simulink model "Q6_c_joint_space_solution"  (R2017a)
settings: Solver=FixedStepAuto  StartTime=0.0  StopTime=10.0  FixedStep=0.01  RelTol=0.00001
model workspace (MAT data in the model file):
  Kp_1 = 10000
  Kp_2 = 10000
  Kv_1 = 200
  Kv_2 = 200
  a_1 = 1
  a_2 = 1
  g = 9.8
  m_1 = 1
  m_2 = 1
  theta_d_dot = 1
  theta_d_double_dot = 1
libraries: simulink x3
settings Model: Creator=Omer  LastModifiedBy=Omer
settings ModelReferenceCC: ModelReferenceMinAlgLoopOccurrences=on

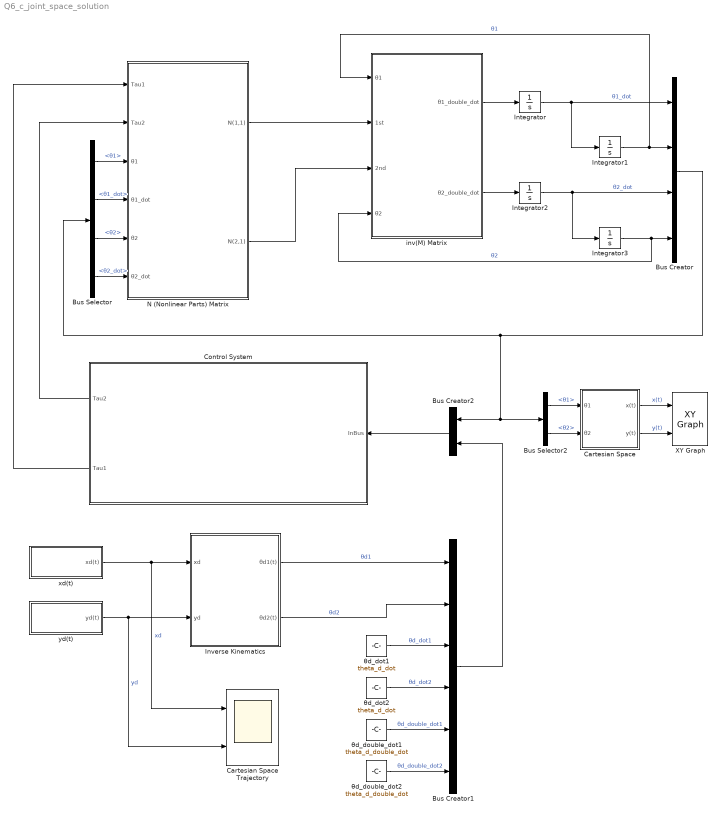
== system Q6_c_joint_space_solution ==
  Bus Creator : BusCreator  Inputs=4
  Bus Creator1 : BusCreator  Inputs=6
  Bus Creator2 : BusCreator  Inputs=2
  Bus Selector : BusSelector  OutputSignals=θ1,θ1_dot,θ2,θ2_dot
  Bus Selector2 : BusSelector  OutputSignals=θ1,θ2
  "Cartesian Space " : Subsystem  TreatAsAtomicUnit=on
  Cartesian Space Trajectory : Scope  NumInputPorts=2
  Control System : Subsystem  TreatAsAtomicUnit=on
  Integrator{,1..3} (4 alike) : Integrator
  Inverse Kinematics : Subsystem  TreatAsAtomicUnit=on
  N (Nonlinear Parts) Matrix : Subsystem  TreatAsAtomicUnit=on
  XY Graph : simulink/Sinks/XY Graph  xmin=-1  xmax=3  ymin=-1  ymax=2  st=-1
  inv(M) Matrix : Subsystem  TreatAsAtomicUnit=on
  xd(t) : Subsystem  TreatAsAtomicUnit=on
  yd(t) : Subsystem  TreatAsAtomicUnit=on
  θd_dot1 : Constant  Value=theta_d_dot
  θd_dot2 : Constant  Value=theta_d_dot
  θd_double_dot1 : Constant  Value=theta_d_double_dot
  θd_double_dot2 : Constant  Value=theta_d_double_dot
  wires:
  N (Nonlinear Parts) Matrix/2(N(2,1)) -> inv(M) Matrix/3(2nd)
  N (Nonlinear Parts) Matrix/1(N(1,1)) -> inv(M) Matrix/2(1st)
  Bus Creator/1 -> Bus Selector2/1, Bus Creator2/1, Bus Selector/1
  inv(M) Matrix/2(θ2_double_dot) -> Integrator2/1
  Bus Selector/1 -> N (Nonlinear Parts) Matrix/3("θ1 ")  "<θ1>"
  Integrator2/1 -> Integrator3/1, Bus Creator/3  "θ2_dot"
  Integrator3/1 -> inv(M) Matrix/4(θ2), Bus Creator/4  "θ2"
  Integrator1/1 -> inv(M) Matrix/1(θ1), Bus Creator/2  "θ1"
  Bus Selector/3 -> N (Nonlinear Parts) Matrix/5(θ2)  "<θ2>"
  Bus Selector/2 -> N (Nonlinear Parts) Matrix/4(θ1_dot)  "<θ1_dot>"
  Integrator/1 -> Bus Creator/1, Integrator1/1  "θ1_dot"
  Bus Selector/4 -> N (Nonlinear Parts) Matrix/6(θ2_dot)  "<θ2_dot>"
  inv(M) Matrix/1(θ1_double_dot) -> Integrator/1
  Bus Selector2/1 -> "Cartesian Space "/1(θ1)  "<θ1>"
  Bus Selector2/2 -> "Cartesian Space "/2(θ2)  "<θ2>"
  "Cartesian Space "/1(x(t)) -> XY Graph/1  "x(t)"
  "Cartesian Space "/2(y(t)) -> XY Graph/2  "y(t)"
  Bus Creator2/1 -> Control System/1(InBus)
  Bus Creator1/1 -> Bus Creator2/2
  θd_dot1/1 -> Bus Creator1/3  "θd_dot1"
  θd_dot2/1 -> Bus Creator1/4  "θd_dot2"
  θd_double_dot1/1 -> Bus Creator1/5  "θd_double_dot1"
  θd_double_dot2/1 -> Bus Creator1/6  "θd_double_dot2"
  xd(t)/1(xd(t)) -> Inverse Kinematics/1(xd), Cartesian Space Trajectory/1  "xd"
  yd(t)/1(yd(t)) -> Inverse Kinematics/2(yd), Cartesian Space Trajectory/2  "yd"
  Control System/1(Tau2) -> N (Nonlinear Parts) Matrix/2(Tau2)
  Control System/2(Tau1) -> N (Nonlinear Parts) Matrix/1(Tau1)
  Inverse Kinematics/1(θd1(t)) -> Bus Creator1/1  "θd1"
  Inverse Kinematics/2(θd2(t)) -> Bus Creator1/2  "θd2"

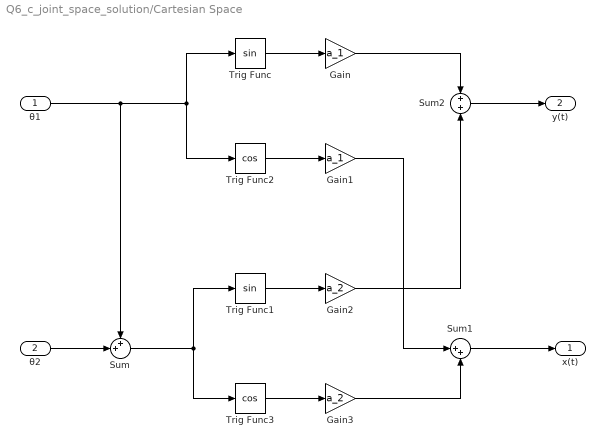
== system Q6_c_joint_space_solution/Cartesian Space  ==
  θ1 : Inport
  θ2 : Inport  Port=2
  Gain : Gain  Gain=a_1
  Gain1 : Gain  Gain=a_1
  Gain2 : Gain  Gain=a_2
  Gain3 : Gain  Gain=a_2
  Sum : Sum  Inputs=++|
  Sum1 : Sum  Inputs=|++
  Sum2 : Sum  Inputs=+|+
  Trig Func : Trigonometry
  Trig Func1 : Trigonometry
  Trig Func2 : Trigonometry  Operator=cos
  Trig Func3 : Trigonometry  Operator=cos
  x(t) : Outport
  y(t) : Outport  Port=2
  wires:
  θ1/1 -> Trig Func2/1, Trig Func/1, Sum/1
  θ2/1 -> Sum/2
  Sum/1 -> Trig Func3/1, Trig Func1/1
  Sum2/1 -> y(t)/1
  Sum1/1 -> x(t)/1
  Trig Func/1 -> Gain/1
  Gain/1 -> Sum2/1
  Trig Func2/1 -> Gain1/1
  Gain1/1 -> Sum1/1
  Trig Func1/1 -> Gain2/1
  Gain2/1 -> Sum2/2
  Trig Func3/1 -> Gain3/1
  Gain3/1 -> Sum1/2

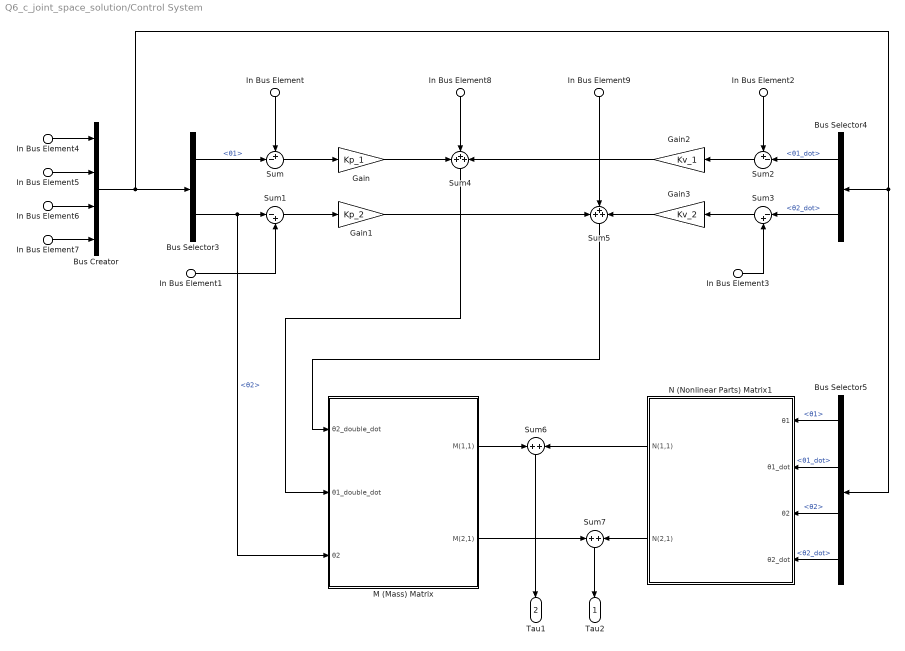
== system Q6_c_joint_space_solution/Control System ==
  In Bus Element : Inport  PortName=InBus  Element=signal2.θd1
  In Bus Element1 : Inport  PortName=InBus  Element=signal2.θd2
  In Bus Element2 : Inport  PortName=InBus  Element=signal2.θd_dot1
  In Bus Element3 : Inport  PortName=InBus  Element=signal2.θd_dot2
  In Bus Element8 : Inport  PortName=InBus  Element=signal2.θd_double_dot1
  In Bus Element9 : Inport  PortName=InBus  Element=signal2.θd_double_dot2
  In Bus Element4 : Inport  PortName=InBus  Element=signal1.θ1_dot
  In Bus Element5 : Inport  PortName=InBus  Element=signal1.θ1
  In Bus Element6 : Inport  PortName=InBus  Element=signal1.θ2_dot
  In Bus Element7 : Inport  PortName=InBus  Element=signal1.θ2
  Bus Creator : BusCreator  Inputs=4
  Bus Selector3 : BusSelector  OutputSignals=θ1,θ2
  Bus Selector4 : BusSelector  OutputSignals=θ1_dot,θ2_dot
  Bus Selector5 : BusSelector  OutputSignals=θ1,θ1_dot,θ2,θ2_dot
  Gain : Gain  Gain=Kp_1
  Gain1 : Gain  Gain=Kp_2
  Gain2 : Gain  Gain=Kv_1
  Gain3 : Gain  Gain=Kv_2
  M (Mass) Matrix : Subsystem  TreatAsAtomicUnit=on
  N (Nonlinear Parts) Matrix1 : Subsystem  TreatAsAtomicUnit=on
  Sum : Sum  Inputs=+-|
  Sum1 : Sum  Inputs=|-+
  Sum2 : Sum  Inputs=+-|
  Sum3 : Sum  Inputs=|-+
  Sum4 : Sum  Inputs=+++
  Sum5 : Sum  Inputs=+++
  Sum6 : Sum  Inputs=+|+
  Sum7 : Sum  Inputs=+|+
  Tau2 : Outport
  Tau1 : Outport  Port=2
  wires:
  Sum4/1 -> M (Mass) Matrix/2(θ1_double_dot)
  M (Mass) Matrix/1(M(1,1)) -> Sum6/1
  In Bus Element1/1 -> Sum1/2
  Sum7/1 -> Tau2/1
  In Bus Element7/1 -> Bus Creator/4
  In Bus Element3/1 -> Sum3/2
  N (Nonlinear Parts) Matrix1/1(N(1,1)) -> Sum6/2
  In Bus Element5/1 -> Bus Creator/2
  Gain1/1 -> Sum5/1
  In Bus Element4/1 -> Bus Creator/1
  Sum3/1 -> Gain3/1
  Sum2/1 -> Gain2/1
  In Bus Element2/1 -> Sum2/1
  Bus Selector5/2 -> N (Nonlinear Parts) Matrix1/2(θ1_dot)  "<θ1_dot>"
  Sum/1 -> Gain/1
  Bus Selector5/3 -> N (Nonlinear Parts) Matrix1/3(θ2)  "<θ2>"
  Sum5/1 -> M (Mass) Matrix/1(θ2_double_dot)
  M (Mass) Matrix/2(M(2,1)) -> Sum7/1
  Bus Selector5/4 -> N (Nonlinear Parts) Matrix1/4(θ2_dot)  "<θ2_dot>"
  Bus Selector4/1 -> Sum2/2  "<θ1_dot>"
  Sum6/1 -> Tau1/1
  Gain/1 -> Sum4/1
  In Bus Element8/1 -> Sum4/2
  In Bus Element9/1 -> Sum5/2
  Bus Selector5/1 -> N (Nonlinear Parts) Matrix1/1("θ1 ")  "<θ1>"
  Gain2/1 -> Sum4/3
  In Bus Element6/1 -> Bus Creator/3
  In Bus Element/1 -> Sum/1
  Gain3/1 -> Sum5/3
  Bus Selector3/2 -> M (Mass) Matrix/3(θ2), Sum1/1  "<θ2>"
  Bus Selector3/1 -> Sum/2  "<θ1>"
  N (Nonlinear Parts) Matrix1/2(N(2,1)) -> Sum7/2
  Bus Selector4/2 -> Sum3/1  "<θ2_dot>"
  Sum1/1 -> Gain1/1
  Bus Creator/1 -> Bus Selector3/1, Bus Selector4/1, Bus Selector5/1

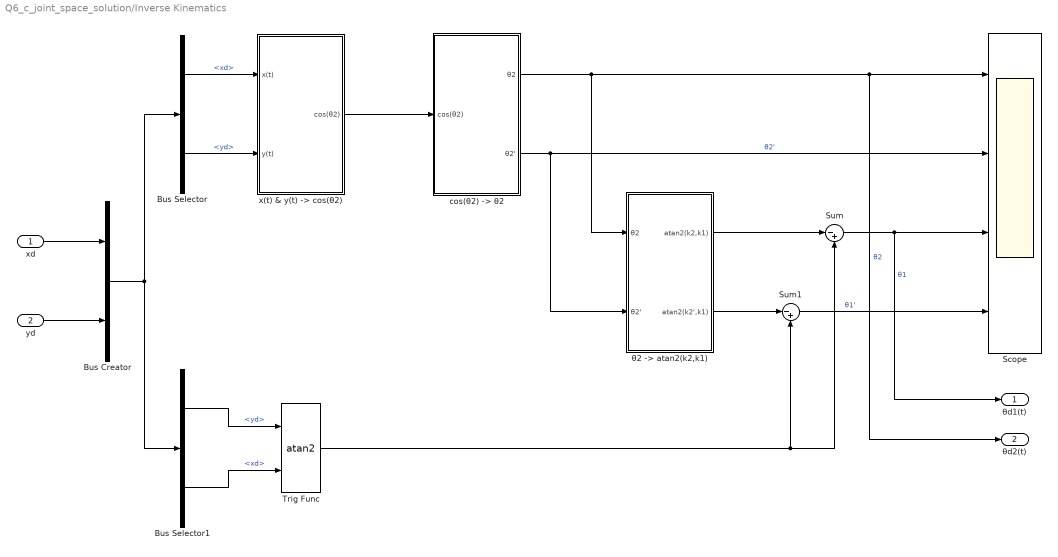
== system Q6_c_joint_space_solution/Inverse Kinematics ==
  xd : Inport
  yd : Inport  Port=2
  Bus Creator : BusCreator  Inputs=2
  Bus Selector : BusSelector  OutputSignals=xd,yd
  Bus Selector1 : BusSelector  OutputSignals=yd,xd
  Scope : Scope  NumInputPorts=4
  Sum : Sum  Inputs=|-+
  Sum1 : Sum  Inputs=|-+
  Trig Func : Trigonometry  Operator=atan2
  "cos(θ2) -> θ2" : Subsystem  TreatAsAtomicUnit=on
  "x(t) & y(t) -> cos(θ2)" : Subsystem  TreatAsAtomicUnit=on
  "θ2 -> atan2(k2,k1) " : Subsystem  TreatAsAtomicUnit=on
  θd1(t) : Outport
  θd2(t) : Outport  Port=2
  wires:
  Sum/1 -> θd1(t)/1, Scope/3  "θ1"
  Bus Selector/1 -> "x(t) & y(t) -> cos(θ2)"/1(x(t))  "<xd>"
  Bus Selector1/1 -> Trig Func/1  "<yd>"
  Sum1/1 -> Scope/4  "θ1'"
  "θ2 -> atan2(k2,k1) "/1(atan2(k2,k1)) -> Sum/1
  "θ2 -> atan2(k2,k1) "/2(atan2(k2',k1)) -> Sum1/1
  "x(t) & y(t) -> cos(θ2)"/1(cos(θ2)) -> "cos(θ2) -> θ2"/1(cos(θ2))
  Bus Selector1/2 -> Trig Func/2  "<xd>"
  Bus Creator/1 -> Bus Selector1/1, Bus Selector/1
  "cos(θ2) -> θ2"/1(θ2) -> "θ2 -> atan2(k2,k1) "/1(θ2), θd2(t)/1, Scope/1  "θ2"
  Bus Selector/2 -> "x(t) & y(t) -> cos(θ2)"/2(y(t))  "<yd>"
  Trig Func/1 -> Sum/2, Sum1/2
  "cos(θ2) -> θ2"/2(θ2') -> "θ2 -> atan2(k2,k1) "/2(θ2'), Scope/2  "θ2'"
  xd/1 -> Bus Creator/1
  yd/1 -> Bus Creator/2

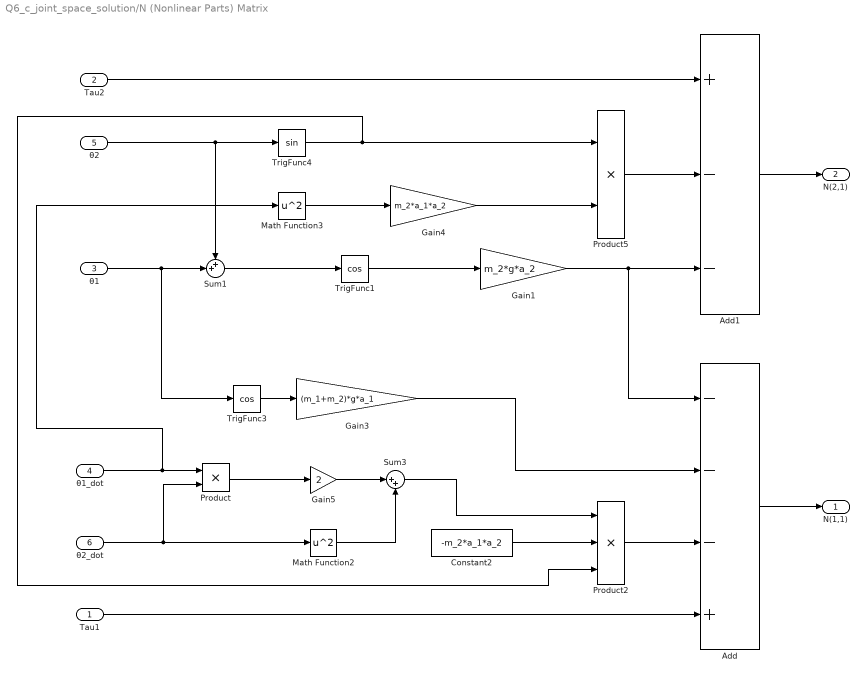
== system Q6_c_joint_space_solution/N (Nonlinear Parts) Matrix ==
  Tau1 : Inport
  Tau2 : Inport  Port=2
  "θ1 " : Inport  Port=3
  θ1_dot : Inport  Port=4
  θ2 : Inport  Port=5
  θ2_dot : Inport  Port=6
  Add : Sum  Inputs=---+
  Add1 : Sum  Inputs=+--
  Constant2 : Constant  Value=-m_2*a_1*a_2
  Gain1 : Gain  Gain=m_2*g*a_2
  Gain3 : Gain  Gain=(m_1+m_2)*g*a_1
  Gain4 : Gain  Gain=m_2*a_1*a_2
  Gain5 : Gain  Gain=2
  Math Function2 : Math  Operator=square  SaturateOnIntegerOverflow=on
  Math Function3 : Math  Operator=square  SaturateOnIntegerOverflow=on
  Product : Product
  Product2 : Product  Inputs=3
  Product5 : Product
  Sum1 : Sum  Inputs=++|
  Sum3 : Sum  Inputs=|++
  TrigFunc1 : Trigonometry  Operator=cos
  TrigFunc3 : Trigonometry  Operator=cos
  TrigFunc4 : Trigonometry
  N(1,1) : Outport
  N(2,1) : Outport  Port=2
  wires:
  Product2/1 -> Add/3
  Gain3/1 -> Add/2
  θ2/1 -> TrigFunc4/1, Sum1/1
  TrigFunc4/1 -> Product2/3, Product5/1
  Add1/1 -> N(2,1)/1
  Math Function3/1 -> Gain4/1
  θ1_dot/1 -> Product/1, Math Function3/1
  θ2_dot/1 -> Product/2, Math Function2/1
  Sum1/1 -> TrigFunc1/1
  Add/1 -> N(1,1)/1
  Sum3/1 -> Product2/1
  Math Function2/1 -> Sum3/2
  Tau2/1 -> Add1/1
  Constant2/1 -> Product2/2
  TrigFunc3/1 -> Gain3/1
  TrigFunc1/1 -> Gain1/1
  "θ1 "/1 -> TrigFunc3/1, Sum1/2
  Product5/1 -> Add1/2
  Tau1/1 -> Add/4
  Gain4/1 -> Product5/2
  Gain1/1 -> Add1/3, Add/1
  Product/1 -> Gain5/1
  Gain5/1 -> Sum3/1

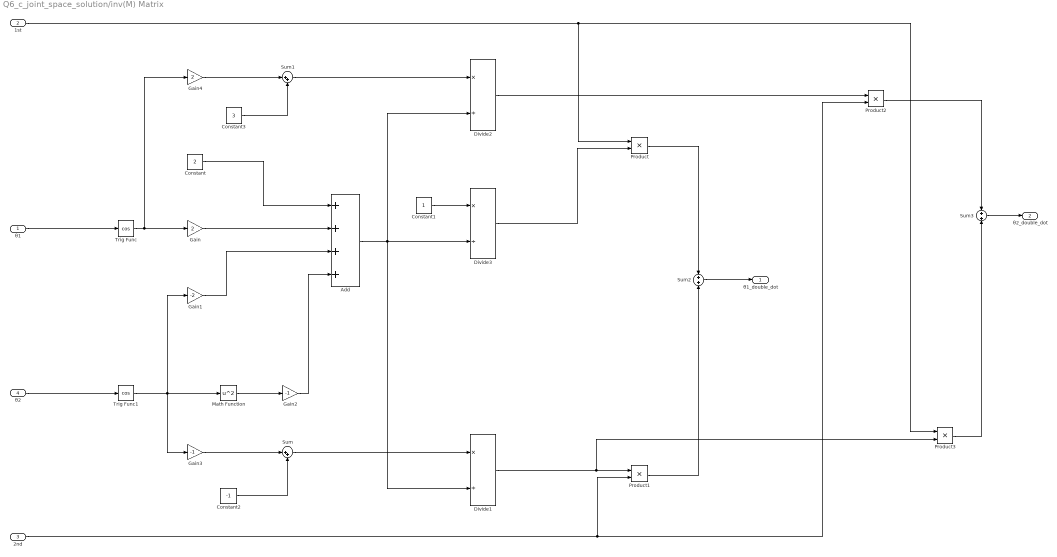
== system Q6_c_joint_space_solution/inv(M) Matrix ==
  θ1 : Inport
  1st : Inport  Port=2
  2nd : Inport  Port=3
  θ2 : Inport  Port=4
  Add : Sum  Inputs=4
  Constant : Constant  Value=2
  Constant1 : Constant
  Constant2 : Constant  Value=-1
  Constant3 : Constant  Value=3
  Divide1 : Product  Inputs=*/
  Divide2 : Product  Inputs=*/
  Divide3 : Product  Inputs=*/
  Gain : Gain  Gain=2
  Gain1 : Gain  Gain=-2
  Gain2 : Gain  Gain=-1
  Gain3 : Gain  Gain=-1
  Gain4 : Gain  Gain=2
  Math Function : Math  Operator=square  SaturateOnIntegerOverflow=on
  Product{,1..3} (4 alike) : Product
  Sum : Sum  Inputs=|++
  Sum1 : Sum  Inputs=|++
  Sum2 : Sum  Inputs=+|+
  Sum3 : Sum  Inputs=+|+
  Trig Func : Trigonometry  Operator=cos
  Trig Func1 : Trigonometry  Operator=cos
  θ1_double_dot : Outport
  θ2_double_dot : Outport  Port=2
  wires:
  Add/1 -> Divide2/2, Divide3/2, Divide1/2
  θ1/1 -> Trig Func/1
  θ2/1 -> Trig Func1/1
  Trig Func1/1 -> Gain3/1, Gain1/1, Math Function/1
  Trig Func/1 -> Gain4/1, Gain/1
  Constant/1 -> Add/1
  Gain/1 -> Add/2
  Gain1/1 -> Add/3
  Constant1/1 -> Divide3/1
  Math Function/1 -> Gain2/1
  Gain2/1 -> Add/4
  Gain3/1 -> Sum/1
  Constant2/1 -> Sum/2
  Sum/1 -> Divide1/1
  Constant3/1 -> Sum1/2
  Gain4/1 -> Sum1/1
  1st/1 -> Product/1, Product3/1
  Divide3/1 -> Product/2
  Divide1/1 -> Product3/2, Product1/1
  2nd/1 -> Product2/2, Product1/2
  Product/1 -> Sum2/1
  Product1/1 -> Sum2/2
  Sum2/1 -> θ1_double_dot/1
  Sum1/1 -> Divide2/1
  Divide2/1 -> Product2/1
  Product2/1 -> Sum3/1
  Sum3/1 -> θ2_double_dot/1
  Product3/1 -> Sum3/2

== system Q6_c_joint_space_solution/xd(t) ==
  Constant : Constant  Value=2
  Product : Product  Inputs=3
  Ramp : simulink/Sources/Ramp  slope=1  start=0  X0=0
  Step : Step  Time=0  SampleTime=0
  Step1 : Step  Time=2  Before=1  After=0  SampleTime=0
  Sum : Sum  Inputs=+-|
  xd(t) : Outport
  wires:
  Product/1 -> xd(t)/1
  Step/1 -> Product/2
  Step1/1 -> Product/3
  Constant/1 -> Sum/1
  Ramp/1 -> Sum/2
  Sum/1 -> Product/1

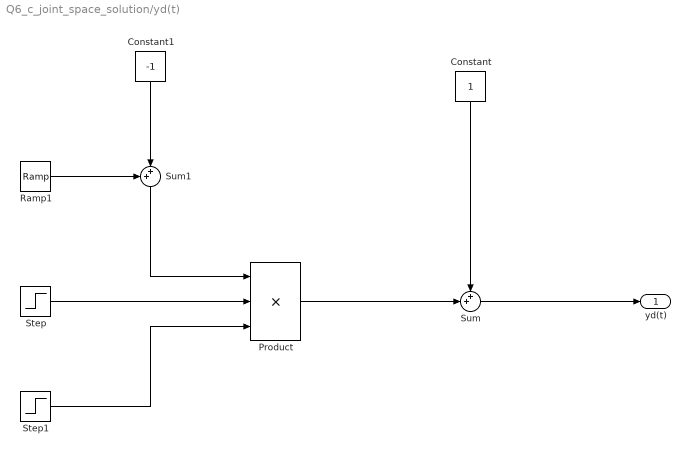
== system Q6_c_joint_space_solution/yd(t) ==
  Constant : Constant
  Constant1 : Constant  Value=-1
  Product : Product  Inputs=3
  Ramp1 : simulink/Sources/Ramp  slope=0.5  start=0  X0=0
  Step : Step  Time=0  SampleTime=0
  Step1 : Step  Time=2  Before=1  After=0  SampleTime=0
  Sum : Sum  Inputs=++|
  Sum1 : Sum  Inputs=++|
  yd(t) : Outport
  wires:
  Step1/1 -> Product/3
  Step/1 -> Product/2
  Sum/1 -> yd(t)/1
  Constant/1 -> Sum/1
  Product/1 -> Sum/2
  Ramp1/1 -> Sum1/1
  Constant1/1 -> Sum1/2
  Sum1/1 -> Product/1

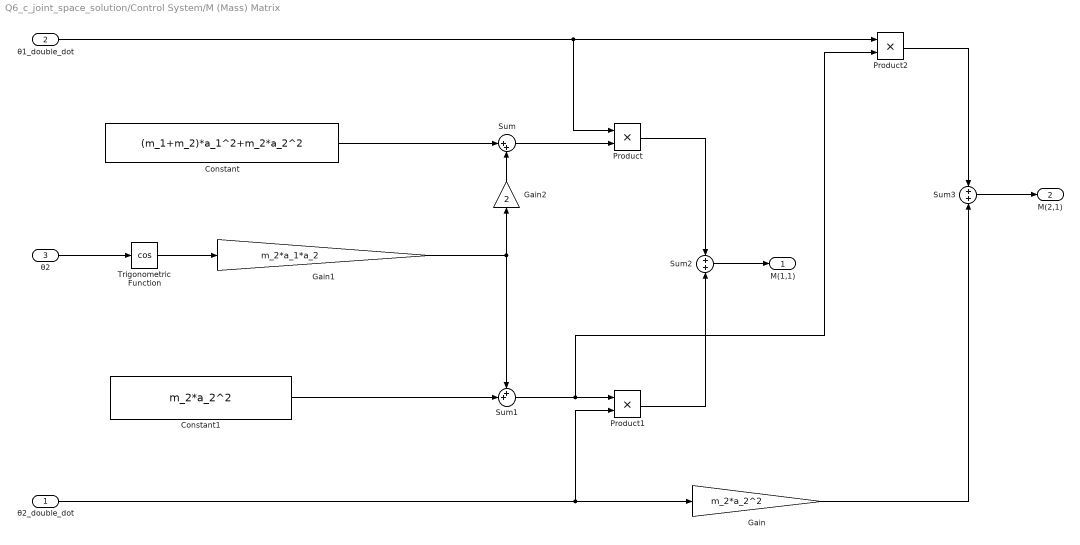
== system Q6_c_joint_space_solution/Control System/M (Mass) Matrix ==
  θ2_double_dot : Inport
  θ1_double_dot : Inport  Port=2
  θ2 : Inport  Port=3
  Constant : Constant  Value=(m_1+m_2)*a_1^2+m_2*a_2^2
  Constant1 : Constant  Value=m_2*a_2^2
  Gain : Gain  Gain=m_2*a_2^2
  Gain1 : Gain  Gain=m_2*a_1*a_2
  Gain2 : Gain  Gain=2
  Product : Product
  Product1 : Product
  Product2 : Product
  Sum : Sum  Inputs=|++
  Sum1 : Sum  Inputs=++|
  Sum2 : Sum  Inputs=+|+
  Sum3 : Sum  Inputs=+|+
  Trigonometric Function : Trigonometry  Operator=cos
  M(1,1) : Outport
  M(2,1) : Outport  Port=2
  wires:
  θ2/1 -> Trigonometric Function/1
  Trigonometric Function/1 -> Gain1/1
  Gain1/1 -> Gain2/1, Sum1/1
  Constant1/1 -> Sum1/2
  Constant/1 -> Sum/1
  θ1_double_dot/1 -> Product/1, Product2/1
  Sum/1 -> Product/2
  Sum1/1 -> Product2/2, Product1/1
  θ2_double_dot/1 -> Gain/1, Product1/2
  Product/1 -> Sum2/1
  Product1/1 -> Sum2/2
  Sum2/1 -> M(1,1)/1
  Product2/1 -> Sum3/1
  Gain/1 -> Sum3/2
  Sum3/1 -> M(2,1)/1
  Gain2/1 -> Sum/2

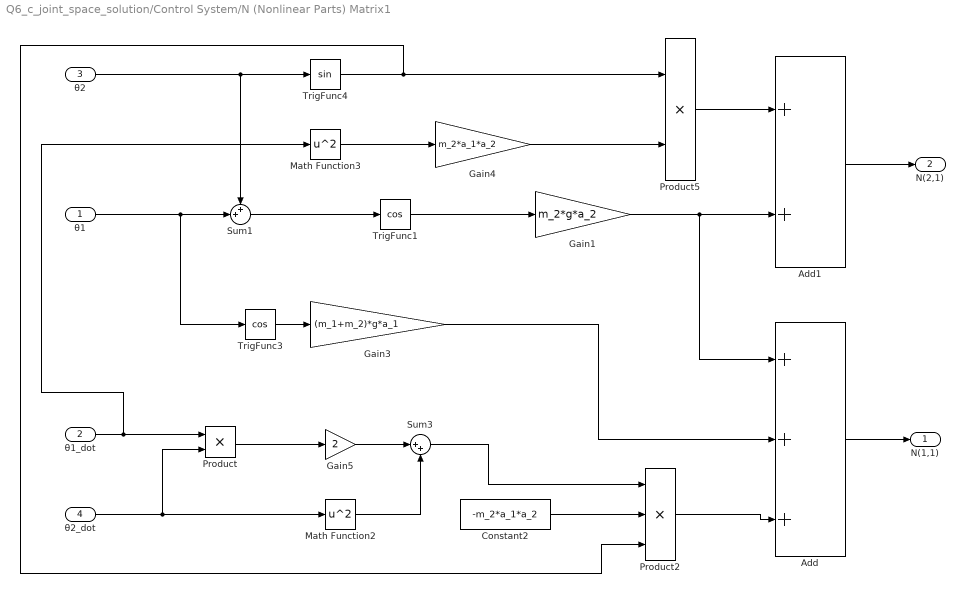
== system Q6_c_joint_space_solution/Control System/N (Nonlinear Parts) Matrix1 ==
  "θ1 " : Inport
  θ1_dot : Inport  Port=2
  θ2 : Inport  Port=3
  θ2_dot : Inport  Port=4
  Add : Sum  Inputs=+++
  Add1 : Sum
  Constant2 : Constant  Value=-m_2*a_1*a_2
  Gain1 : Gain  Gain=m_2*g*a_2
  Gain3 : Gain  Gain=(m_1+m_2)*g*a_1
  Gain4 : Gain  Gain=m_2*a_1*a_2
  Gain5 : Gain  Gain=2
  Math Function2 : Math  Operator=square  SaturateOnIntegerOverflow=on
  Math Function3 : Math  Operator=square  SaturateOnIntegerOverflow=on
  Product : Product
  Product2 : Product  Inputs=3
  Product5 : Product
  Sum1 : Sum  Inputs=++|
  Sum3 : Sum  Inputs=|++
  TrigFunc1 : Trigonometry  Operator=cos
  TrigFunc3 : Trigonometry  Operator=cos
  TrigFunc4 : Trigonometry
  N(1,1) : Outport
  N(2,1) : Outport  Port=2
  wires:
  Product2/1 -> Add/3
  Gain3/1 -> Add/2
  θ2/1 -> TrigFunc4/1, Sum1/1
  TrigFunc4/1 -> Product2/3, Product5/1
  Add1/1 -> N(2,1)/1
  Math Function3/1 -> Gain4/1
  θ1_dot/1 -> Product/1, Math Function3/1
  θ2_dot/1 -> Product/2, Math Function2/1
  Sum1/1 -> TrigFunc1/1
  Add/1 -> N(1,1)/1
  Sum3/1 -> Product2/1
  Math Function2/1 -> Sum3/2
  Constant2/1 -> Product2/2
  TrigFunc3/1 -> Gain3/1
  TrigFunc1/1 -> Gain1/1
  "θ1 "/1 -> TrigFunc3/1, Sum1/2
  Gain4/1 -> Product5/2
  Gain1/1 -> Add/1, Add1/2
  Product/1 -> Gain5/1
  Gain5/1 -> Sum3/1
  Product5/1 -> Add1/1

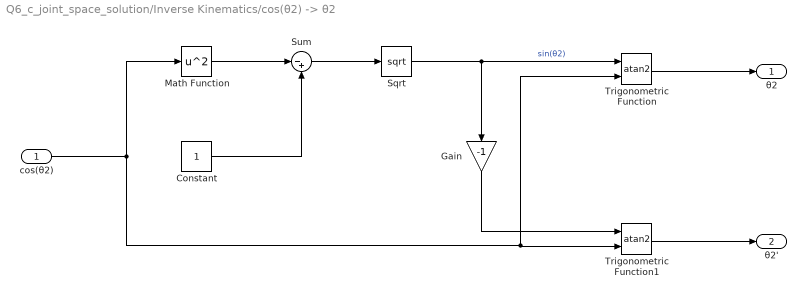
== system Q6_c_joint_space_solution/Inverse Kinematics/cos(θ2) -> θ2 ==
  cos(θ2) : Inport
  Constant : Constant
  Gain : Gain  Gain=-1
  Math Function : Math  Operator=square  SaturateOnIntegerOverflow=on
  Sqrt : Sqrt  SaturateOnIntegerOverflow=on
  Sum : Sum  Inputs=|-+
  Trigonometric Function : Trigonometry  Operator=atan2
  Trigonometric Function1 : Trigonometry  Operator=atan2
  θ2 : Outport
  θ2' : Outport  Port=2
  wires:
  cos(θ2)/1 -> Trigonometric Function/2, Trigonometric Function1/2, Math Function/1
  Math Function/1 -> Sum/1
  Constant/1 -> Sum/2
  Sum/1 -> Sqrt/1
  Sqrt/1 -> Gain/1, Trigonometric Function/1  "sin(θ2)"
  Trigonometric Function/1 -> θ2/1
  Trigonometric Function1/1 -> θ2'/1
  Gain/1 -> Trigonometric Function1/1

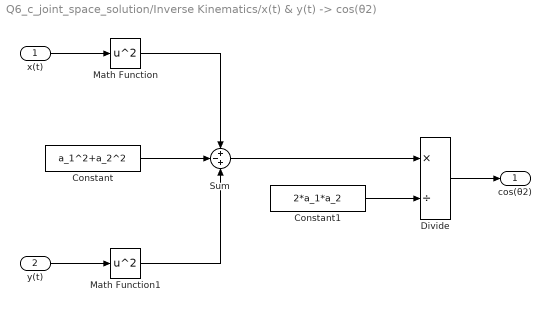
== system Q6_c_joint_space_solution/Inverse Kinematics/x(t) & y(t) -> cos(θ2) ==
  x(t) : Inport
  y(t) : Inport  Port=2
  Constant : Constant  Value=a_1^2+a_2^2
  Constant1 : Constant  Value=2*a_1*a_2
  Divide : Product  Inputs=*/
  Math Function : Math  Operator=square  SaturateOnIntegerOverflow=on
  Math Function1 : Math  Operator=square  SaturateOnIntegerOverflow=on
  Sum : Sum  Inputs=+-+
  cos(θ2) : Outport
  wires:
  x(t)/1 -> Math Function/1
  y(t)/1 -> Math Function1/1
  Math Function/1 -> Sum/1
  Constant/1 -> Sum/2
  Math Function1/1 -> Sum/3
  Divide/1 -> cos(θ2)/1
  Sum/1 -> Divide/1
  Constant1/1 -> Divide/2

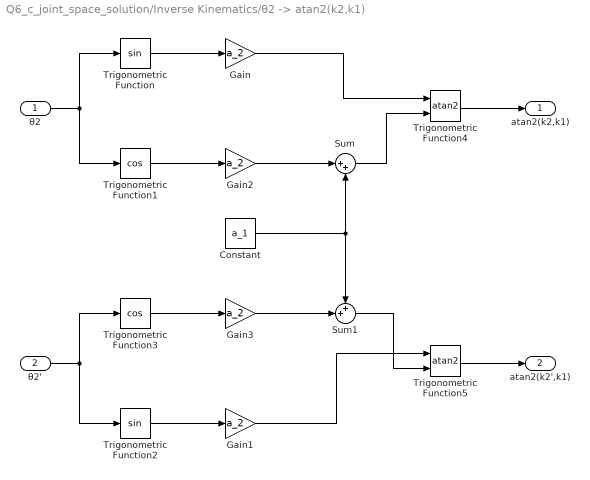
== system Q6_c_joint_space_solution/Inverse Kinematics/θ2 -> atan2(k2,k1)  ==
  θ2 : Inport
  θ2' : Inport  Port=2
  Constant : Constant  Value=a_1
  Gain{,1..3} (4 alike) : Gain  Gain=a_2
  Sum : Sum  Inputs=|++
  Sum1 : Sum  Inputs=++|
  Trigonometric Function : Trigonometry
  Trigonometric Function1 : Trigonometry  Operator=cos
  Trigonometric Function2 : Trigonometry
  Trigonometric Function3 : Trigonometry  Operator=cos
  Trigonometric Function4 : Trigonometry  Operator=atan2
  Trigonometric Function5 : Trigonometry  Operator=atan2
  atan2(k2,k1) : Outport
  atan2(k2',k1) : Outport  Port=2
  wires:
  θ2/1 -> Trigonometric Function/1, Trigonometric Function1/1
  θ2'/1 -> Trigonometric Function2/1, Trigonometric Function3/1
  Trigonometric Function/1 -> Gain/1
  Trigonometric Function1/1 -> Gain2/1
  Trigonometric Function3/1 -> Gain3/1
  Trigonometric Function2/1 -> Gain1/1
  Gain2/1 -> Sum/1
  Constant/1 -> Sum1/1, Sum/2
  Gain1/1 -> Trigonometric Function5/1
  Gain/1 -> Trigonometric Function4/1
  Sum/1 -> Trigonometric Function4/2
  Trigonometric Function4/1 -> atan2(k2,k1)/1
  Trigonometric Function5/1 -> atan2(k2',k1)/1
  Gain3/1 -> Sum1/2
  Sum1/1 -> Trigonometric Function5/2
